simulink model "Lab_2_model"  (R2024a)
settings: Solver=VariableStepAuto  StartTime=0.0  StopTime=100  MaxStep=0.01  RelTol=1e-4  EnableMultiTasking=on
undefined symbols (not defined in the file or in its folder): den, gain, num
settings Model: Creator=Zwivh  LastModifiedBy=Zwivh
settings SolverCC: AlgebraicLoopSolver=TrustRegion
settings DataIOCC: LimitDataPoints=on  SaveOutput=off  SaveTime=off
settings OptimizationCC: ExpressionDepthLimit=2147483647  LifeSpan=1
settings DebuggingCC: UnderspecifiedInitializationDetection=Classic  MergeDetectMultiDrivingBlocksExec=none  FcnCallInpInsideContextMsg=warning  UnconnectedInputMsg=warning  UnconnectedOutputMsg=warning  UnconnectedLineMsg=warning  AllowSymbolicDim=off  StateNameClashWarn=warning  SFUnexpectedBacktrackingDiag=warning  SFNoUnconditionalDefaultTransitionDiag=warning  SFExecutionAtInitializationDiag=none  ArithmeticOperatorsInVariantConditions=warning
settings ModelReferenceCC: EnableRefExpFcnMdlSchedulingChecks=on
settings SFSimCC: SimUseLocalCustomCode=off  CustomCodeUndefinedFunction=UseInterfaceOnly
settings RTWCC: RTWUseLocalCustomCode=off  GPUComputeCapability=3.5
settings CodeAppCC: StateflowObjectComments=on
settings GRTTargetCC: TargetLangStandard=C89/C90 (ANSI)  CombineOutputUpdateFcns=off  GRTInterface=on

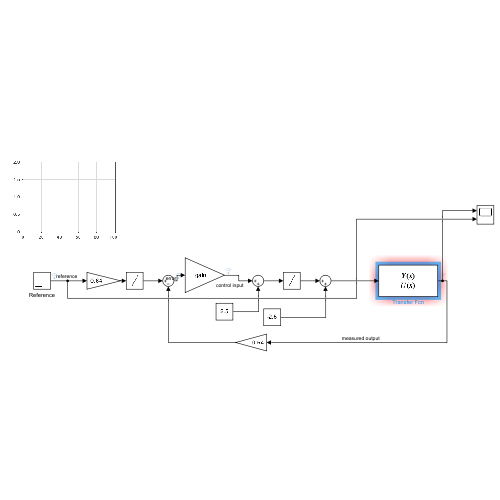
[thumbnail: Simulink's stored preview of the top-level diagram]
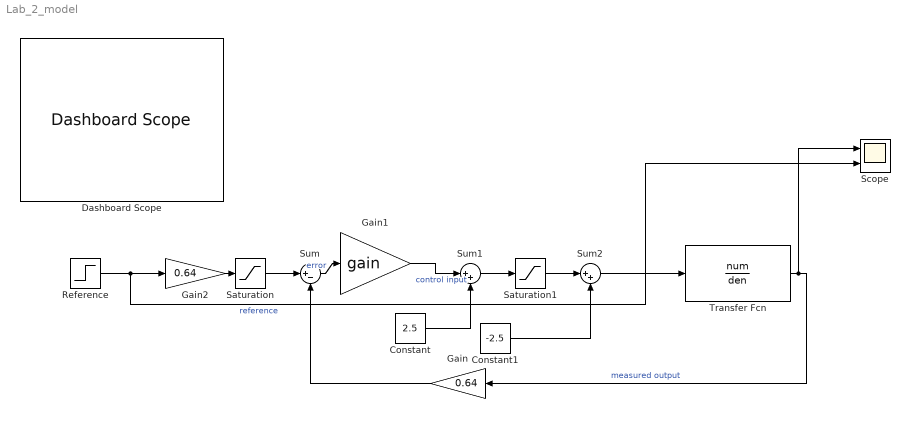
== system Lab_2_model ==
  Constant : Constant  Value=2.5
  Constant1 : Constant  Value=-2.5
  Dashboard Scope : DashboardScope  Ymin=0  Ymax=2  NormalizeYAxis=on
  Gain : Gain  Gain=0.64
  Gain1 : Gain  Gain=gain
  Gain2 : Gain  Gain=0.64
  Reference : Step  SampleTime=0
  Saturation : Saturate  UpperLimit=5  LowerLimit=0
  Saturation1 : Saturate  UpperLimit=5  LowerLimit=0
  Scope : Scope  NumInputPorts=2
  Sum : Sum  Inputs=|+-
  Sum1 : Sum  Inputs=|++
  Sum2 : Sum  Inputs=|++
  Transfer Fcn : TransferFcn  Numerator=num  Denominator=den
  wires:
  Reference/1 -> Scope/2, Gain2/1  "reference"
  Transfer Fcn/1 -> Gain/1, Scope/1  "measured output"
  Sum/1 -> Gain1/1  "error"
  Gain/1 -> Sum/2
  Gain1/1 -> Sum1/1  "control input"
  Constant/1 -> Sum1/2
  Constant1/1 -> Sum2/2
  Gain2/1 -> Saturation/1
  Saturation/1 -> Sum/1
  Saturation1/1 -> Sum2/1
  Sum2/1 -> Transfer Fcn/1
  Sum1/1 -> Saturation1/1
